simulink model "encoder"  (R2015b)
settings: Solver=VariableStepAuto  StartTime=0.0  StopTime=inf  RelTol=1e-3
libraries: realtime_pacer_lib x1, robotlib x1
settings Model: Creator=rotem  LastModifiedBy=saucer

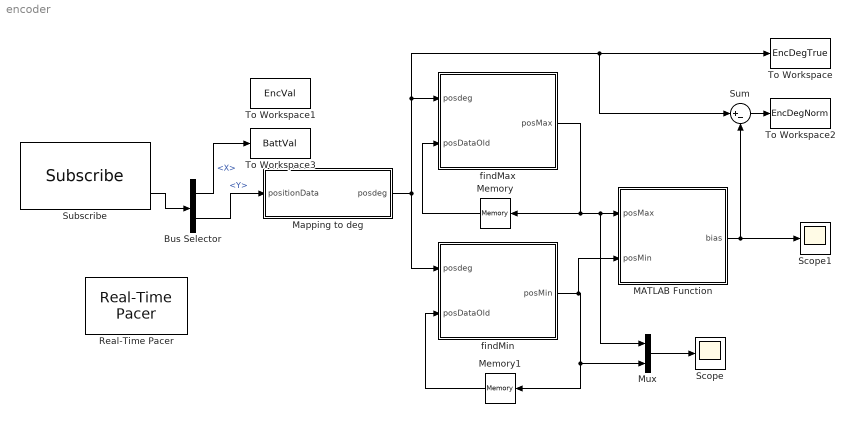
== system encoder ==
  Bus Selector : BusSelector  OutputSignals=X,Y
  MATLAB Function : MATLAB Function  TreatAsAtomicUnit=on
  Mapping to deg : MATLAB Function  TreatAsAtomicUnit=on
  Memory : Memory  X0=-360
  Memory1 : Memory  X0=360
  Mux : Mux  Inputs=2
  Real-Time Pacer : realtime_pacer_lib/Real-Time Pacer  simTimePerRealTime=1
  Scope : Scope
  Scope1 : Scope
  Subscribe : robotlib/Subscribe  SourceLibraryInfo=This block requires Robotics System Toolbox  topicSource=Select from ROS network  topic=/BatteryAndEncoder  messageType=geometry_msgs/Vector3  sampleTime=-1  messageQueueLength=1
  Sum : Sum  Inputs=|+-
  To Workspace : ToWorkspace  VariableName=EncDegTrue  SaveFormat=Timeseries  SampleTime=-1
  To Workspace1 : ToWorkspace  VariableName=EncVal  SaveFormat=Timeseries  SampleTime=-1
  To Workspace2 : ToWorkspace  VariableName=EncDegNorm  SaveFormat=Timeseries  SampleTime=-1
  To Workspace3 : ToWorkspace  VariableName=BattVal  SaveFormat=Timeseries  SampleTime=-1
  findMax : MATLAB Function  TreatAsAtomicUnit=on
  findMin : MATLAB Function  TreatAsAtomicUnit=on
  wires:
  Subscribe/2 -> Bus Selector/1
  findMax/1(posMax) -> Memory/1, Mux/1, MATLAB Function/1(posMax)
  Memory/1 -> findMax/2(posDataOld)
  Mapping to deg/1(posdeg) -> Sum/1, To Workspace/1, findMax/1(posdeg), findMin/1(posdeg)
  findMin/1(posMin) -> MATLAB Function/2(posMin), Mux/2, Memory1/1
  Memory1/1 -> findMin/2(posDataOld)
  MATLAB Function/1(bias) -> Scope1/1, Sum/2
  Sum/1 -> To Workspace2/1
  Mux/1 -> Scope/1
  Bus Selector/2 -> Mapping to deg/1(positionData)  "<Y>"
  Bus Selector/1 -> To Workspace3/1  "<X>"

== matlab function encoder/findMax ==
  data: posdeg input; posMax output; posDataOld input
function posMax = findMax(posdeg,posDataOld)
posMax = posDataOld;
if posdeg > posDataOld
    posMax = posdeg;
end

== matlab function encoder/Mapping to deg ==
  data: positionData input; posdeg output
function posdeg = val2deg(positionData)
%#codegen
puls = 2*2048; %2 channels x 2048 CPR
degpp = 360/puls; %Degrees pr. pulse.
% positionData = uint32(positionData); %Convert from double to uint32

%Convertion to signed data:
counterNBits = 12; %Bits in the encoder reading
signedThreshold = 2^(counterNBits-1); %Treshold for convertion to signed pos. values
signedData = positionData;
signedData(signedData > signedThreshold) = signedData(signedData > signedThreshold) - 2^counterNBits;

posdeg = signedData*degpp;

== matlab function encoder/findMin ==
  data: posdeg input; posMin output; posDataOld input
function posMin = findMin(posdeg,posDataOld)
posMin = posDataOld;
if posdeg < posDataOld
    posMin = posdeg;
end

== matlab function encoder/MATLAB Function ==
  data: posMax input; bias output; posMin input
function bias = normalRange(posMax,posMin)
range = posMax-posMin;
bias = posMin + range/2;
